simulink model "QUESTION3"  (R2020a)
settings: Solver=VariableStepAuto  StartTime=0.0  StopTime=10.0  RelTol=1e-3
model workspace (MAT data in the model file):
  b = Simulink.Parameter
  b.Value = 50
  b.DataType = 'auto'
  b.Dimensions = [1 1]
  ki = Simulink.Parameter
  ki.Value = 300
  ki.DataType = 'auto'
  ki.Dimensions = [1 1]
  kp = Simulink.Parameter
  kp.Value = 350
  kp.DataType = 'auto'
  kp.Dimensions = [1 1]
  m = Simulink.Parameter
  m.Value = 1000
  m.DataType = 'auto'
  m.Dimensions = [1 1]
  u = Simulink.Parameter
  u.Value = 500
  u.DataType = 'auto'
  u.Dimensions = [1 1]
settings Model: OrderedModelArguments=off  Creator=anjal  LastModifiedBy=anjal

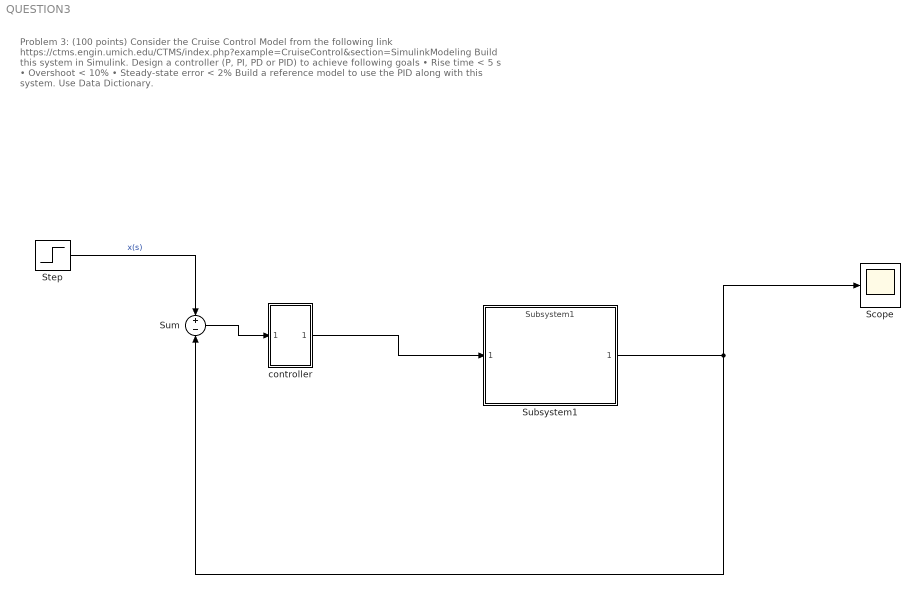
== system QUESTION3 ==
  note: Problem 3: (100 points) Consider the Cruise Control Model from the following link
      | https://ctms.engin.umich.edu/CTMS/index.php?example=CruiseControl&section=SimulinkModeling Build this system in Simulink.
      | Design a controller (P, PI, PD or PID) to achieve following goals
      | • Rise time < 5 s
      | • Overshoot < 10%
      | • Steady-state error < 2%
      | Build a reference model to use the PID along with this system. Use Data Dictionary.
  Scope : Scope
  Step : Step  Time=0  After=u  SampleTime=0
  Subsystem1 : ModelReference  ModelNameDialog=Subsystem1  ModelReferenceVersion=1.17
  Sum : Sum  Inputs=+-
  controller : Subsystem
  wires:
  Step/1 -> Sum/1  "x(s)"
  Sum/1 -> controller/1(In1)
  Subsystem1/1 -> Scope/1, Sum/2
  controller/1(Out1) -> Subsystem1/1

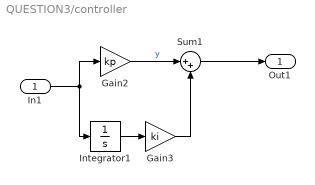
== system QUESTION3/controller ==
  In1 : Inport
  Gain2 : Gain  Gain=kp
  Gain3 : Gain  Gain=ki
  Integrator1 : Integrator
  Sum1 : Sum  Inputs=|++
  Out1 : Outport
  wires:
  Integrator1/1 -> Gain3/1
  In1/1 -> Integrator1/1, Gain2/1
  Sum1/1 -> Out1/1
  Gain3/1 -> Sum1/2
  Gain2/1 -> Sum1/1  "y"
